simulink model "Serialsend_position"  (R2020a)
settings: Solver=ode4  StartTime=0.0  StopTime=10  FixedStep=0.002  RelTol=1e-3
undefined symbols (not defined in the file): LF, serial
libraries: instrumentlib x2
settings Model: EnablePacing=on  Creator=shiib  LastModifiedBy=Natsu Nakagawa
settings DataIOCC: ReturnWorkspaceOutputs=off
settings DebuggingCC: ArithmeticOperatorsInVariantConditions=warning
settings SFSimCC: SimUseLocalCustomCode=off  CustomCodeUndefinedFunction=UseInterfaceOnly
settings RTWCC: RTWUseLocalCustomCode=off

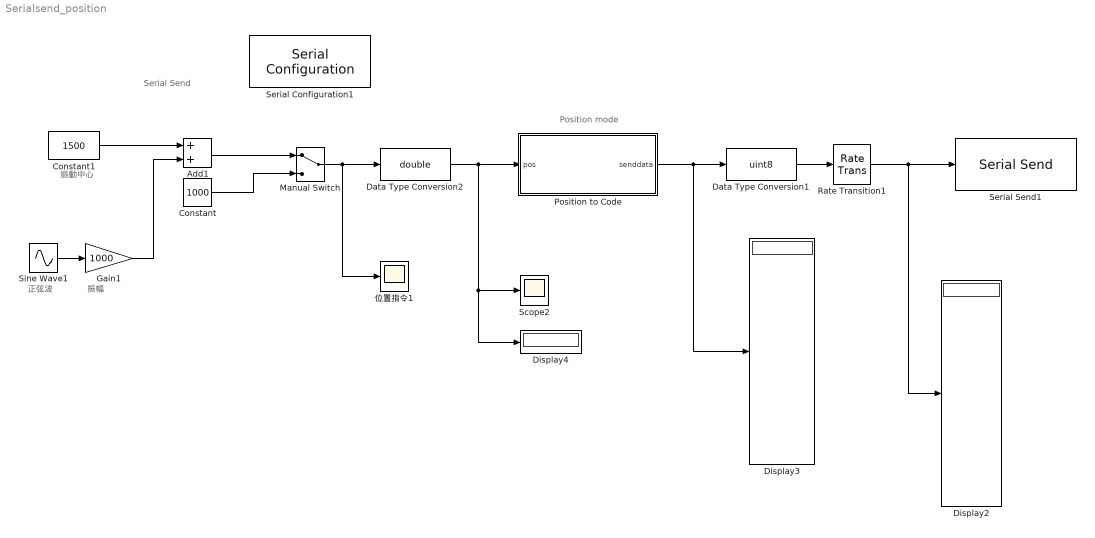
== system Serialsend_position ==
  note: Position mode
  note: Serial Send
  note: 振動中心
  note: 正弦波
  note: 振幅
  Add1 : Sum
  Constant : Constant  Value=1000
  Constant1 : Constant  Value=1500  OutDataTypeStr=int16  SampleTime=1
  Data Type Conversion1 : DataTypeConversion  OutDataTypeStr=uint8
  Data Type Conversion2 : DataTypeConversion  OutDataTypeStr=double  RndMeth=Ceiling
  Display2 : Display
  Display3 : Display
  Display4 : Display
  Gain1 : Gain  Gain=1000  OutDataTypeStr=int16
  Manual Switch : ManualSwitch
  Position to Code : MATLAB Function  TreatAsAtomicUnit=on
  Rate Transition1 : RateTransition  OutPortSampleTime=0.004
  Scope2 : Scope
  Serial Configuration1 : instrumentlib/Serial Configuration  Priority=-200000  ComPortMenu=<Please select a port...>  ComPort=/dev/cu.usbserial-FTS6VUOQ  ObjConstructor=serial('/dev/cu.usbserial-FTS6VUOQ');  BaudRate=115200  DataBits=8  Parity=none  StopBits=1  FlowControl=none  Timeout=10  ByteOrder=LittleEndian
  Serial Send1 : instrumentlib/Serial Send  ComPortMenu=<Please select a port...>  ComPort=/dev/cu.usbserial-FTS6VUOQ  ObjConstructor=serial('/dev/cu.usbserial-FTS6VUOQ');  Terminator=LF ('\n')  EnableBlockingMode=on
  Sine Wave1 : Sin  Frequency=3.14  SampleTime=0
  位置指令1 : Scope
  wires:
  Data Type Conversion1/1 -> Rate Transition1/1
  Data Type Conversion2/1 -> Position to Code/1(pos), Scope2/1, Display4/1
  Position to Code/1(senddata) -> Data Type Conversion1/1, Display3/1
  Constant1/1 -> Add1/1
  Sine Wave1/1 -> Gain1/1
  Gain1/1 -> Add1/2
  Manual Switch/1 -> 位置指令1/1, Data Type Conversion2/1
  Add1/1 -> Manual Switch/1
  Constant/1 -> Manual Switch/2
  Rate Transition1/1 -> Serial Send1/1, Display2/1

== matlab function Serialsend_position/Position to Code ==
  data: pos input; senddata output
% script_sendTargetPosition
% MATLAB EPOS LibraryのsendTargetPosition()から書き換え

% function [] = sendTargetPosition( obj, pos )

function senddata = func_sendTargetPosition(pos)
%Sets the TargetPosition for Profile Position mode
%pos must be an integer.
pos_hex = '';

if pos >= 0
    pos_hex = dec2hex(pos, 8);
else
    pos_hex = dec2hex(2^32+pos, 8);
end

%% Build write object request frame EPOS Node 1
%SYNC: The first two bytes are used for frame synchronization.(EPOS4)
%   “DLE” (Data Link Escape) = 0x90
%   “STX” (Start of Text) = 0x02
DLE = uint16(0x90);
STX = uint16(0x02);

%HEADER: The header consists of 2 bytes. The first field determines the type of data frame to be sent or received. The next field contains the length of the data fields.
%   "OpCode"(write) = 0x68
%   "Len" = 0x04
OpCode = uint16(0x68);
Len = uint16(0x04);

%DATA: The data fields contain the parameters of the message. The low byte of the word is transmitted first.
%   NodeID = 0x01
%   Index of Object (Target Position): 0x607A
%   Subindex of Object = 0x00
%   Data byte to write[4]: pos_hex(1:4), pos_hex(5:8)
DATA = uint16([0x01 0x7A 0x60 0x00 myhex2dec(pos_hex(7:8)) myhex2dec(pos_hex(5:6)) myhex2dec(pos_hex(3:4)) myhex2dec(pos_hex(1:2))])

%DATAforCRC
%   uint16([myhex2dec('6804') myhex2dec('2062') myhex2dec('0100') myhex2dec(pos_hex(5:8)) myhex2dec(pos_hex(1:4)) myhex2dec('0000')]);
DATAforCRC = uint16([0x0468 0x7A01 0x0060 myhex2dec(pos_hex(5:8)) myhex2dec(pos_hex(1:4)) 0x0000]);
numberofWordsCRC = Len+2;
crc_hex = dec2hex(CRCcalc(DATAforCRC, numberofWordsCRC),4);
CRC = uint16([myhex2dec(crc_hex(3:4)) myhex2dec(crc_hex(1:2))]);

% senddata=[opCode Len_1 DATA CRC char('O')];
% senddata=[opCode Len_1 DATA CRC 79 10]';
senddata=[DLE STX OpCode Len DATA CRC]';

end


function d = myhex2dec(h)
%HEX2DEC Convert hexadecimal string to decimal integer.
%   this is the hex2dec function from Matlab with some checking disabled
%   for faster performance

if iscellstr(h), h = char(h); end
if isempty(h), d = []; return, end

% Work in upper case. - disabled since upper case anyways
%h = upper(h);

[m,n]=size(h);

% Right justify strings and form 2-D character array.
if ~isempty(find((h==' ' | h==0),1))
  h = strjust(h);

  % Replace any leading blanks and nulls by 0.
  h(cumsum(h ~= ' ' & h ~= 0,2) == 0) = '0';
else
  h = reshape(h,m,n);
end

% Check for out of range values - disabled
% if any(any(~((h>='0' & h<='9') | (h>='A'&h<='F'))))
%    error(message('MATLAB:hex2dec:IllegalHexadecimal'));
% end

sixteen = 16;
p = fliplr(cumprod([1 sixteen(ones(1,n-1))]));
p = p(ones(m,1),:);

d = h <= 64; % Numbers
h(d) = h(d) - 48;

d =  h > 64; % Letters
h(d) = h(d) - 55;

d = sum(h.*p,2);


end

function [ CRC ] = CRCcalc(DataArray, CRCnumberOfWords)
%Calculates the 16 bit CRC checksum according to communication guide for
%EPOS2
%Arguments are the DataArray that is being sent (opCode to Data) and the
%number of words

CRC = uint16(0);
for i=1:CRCnumberOfWords
    
    %shifter = uint16(myhex2dec('8000'));
    shifter = uint16(32768);
    c = DataArray(i);
    
    while(shifter)
        %carry = bitand(CRC, uint16(myhex2dec('8000')), 'uint16');
        carry = bitand(CRC, uint16(32768), 'uint16');
        CRC = bitshift(CRC,1,'uint16');
        if(bitand(c, shifter, 'uint16'))
            CRC = CRC +  1;
        end
        if(carry)
            %CRC = bitxor(CRC,uint16(myhex2dec('1021')),'uint16');
            CRC = bitxor(CRC,uint16(4129),'uint16');
        end
        shifter = bitshift(shifter,-1,'uint16');
    end
    
end


end
